simulink model "gm_uz_endat_interface_2023a"  (R2023a)
settings: Solver=FixedStepDiscrete  StartTime=0.0  StopTime=1.3e-3  RelTol=1e-3
undefined symbols (not defined in the file or in its folder): binary_or_gray, bit_sum, delay_first_clk_on_off, endat_clk_divider, endat_encoder_bit_width_multi_turn, endat_encoder_bit_width_single_turn, endat_encoder_number_of_CRC_bits, f_ADC, f_clock, PLL, t_ADC, t_clock
libraries: hdlmdlgenlib x127, simulink x35, hdlsllib x24, simulink_extras x12
(part 1 of 4)
settings Model: Creator=micha  LastModifiedBy=micha
settings SolverCC: AlgebraicLoopSolver=TrustRegion
settings DataIOCC: LimitDataPoints=on  SaveOutput=off  SaveTime=off
settings OptimizationCC: BlockReduction=off  ConditionallyExecuteInputs=off  DefaultParameterBehavior=Inlined  InheritOutputTypeSmallerThanSingle=on  LifeSpan=inf
settings DebuggingCC: AlgebraicLoopMsg=error  ArtificialAlgebraicLoopMsg=none  InheritedTsInSrcMsg=none  SingleTaskRateTransMsg=error  UnconnectedInputMsg=warning  UnconnectedOutputMsg=warning  UnconnectedLineMsg=warning  AllowSymbolicDim=off  StrictBusMsg=ErrorOnBusTreatedAsVector  SFUnexpectedBacktrackingDiag=warning  SFNoUnconditionalDefaultTransitionDiag=warning  SFExecutionAtInitializationDiag=none  ArithmeticOperatorsInVariantConditions=warning
settings HardwareCC: ProdBitPerPointer=32  ProdBitPerSizeT=32  ProdBitPerPtrDiffT=32  ProdLargestAtomicFloat=None  ProdIntDivRoundTo=Undefined  ProdEndianess=Unspecified  ProdWordSize=32  ProdHWDeviceType=ASIC/FPGA->ASIC/FPGA  ProdEqTarget=off
settings ModelReferenceCC: EnableRefExpFcnMdlSchedulingChecks=on
settings SFSimCC: SimUseLocalCustomCode=off  CustomCodeUndefinedFunction=UseInterfaceOnly
settings RTWCC: RTWUseLocalCustomCode=off  DLArmComputeVersion=19.05
settings CodeAppCC: StateflowObjectComments=on
settings GRTTargetCC: TargetLangStandard=C89/C90 (ANSI)
settings ConfigComp: CovScope=ReferencedModels  CovMetricSettings=dw  CovSaveCumulativeToWorkspaceVar=on  CovSaveSingleToWorkspaceVar=on  CovExternalEMLEnable=off  CovSFcnEnable=off

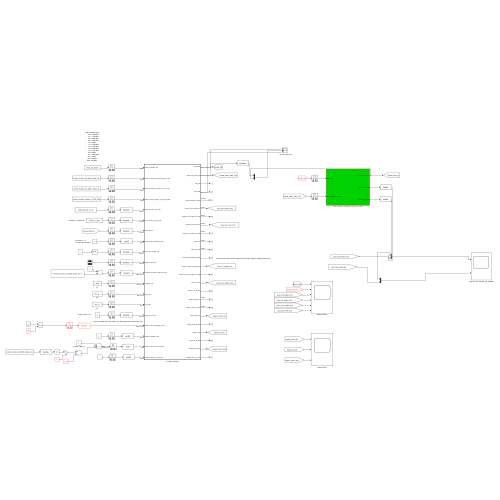
[thumbnail: Simulink's stored preview of the top-level diagram]
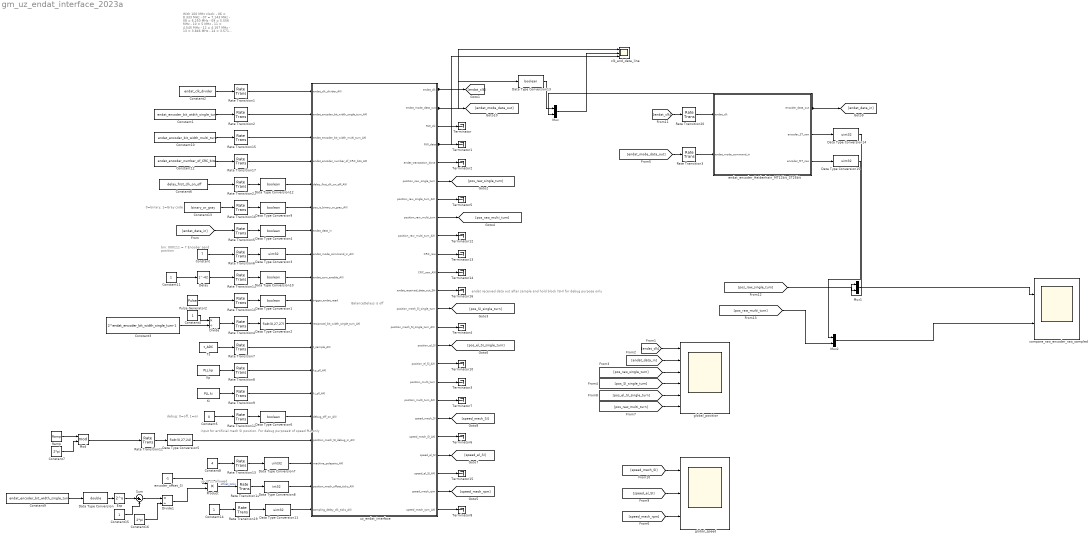
== system gm_uz_endat_interface_2023a ==
  note: 0=binary, 1=Gray code
  note: With 100 MHz clock:
      | -     06 = 8.333 MHz
      | -     07 = 7.143 MHz
      | -     08 = 6.250 MHz
      | -     09 = 5.556 MHz
      | -     10 = 5 MHz
      | -     11 = 4.545 MHz
      | -     12 = 4.167 MHz
      | -     13 = 3.846 MHz
      | -     14 = 3.571 MHz
      | -     25 = 2 MHz
      | -     27 = 1.852 MHz
      | -     50 = 1 MHz
      | -   100 = 500 kHz
      | -   200 = 250 kHz
  note: BalanceDelays is off
  note: debug: 0=off, 1=on
  note: up to 21 allowed
  note: endat received data out after sample and hold block (SH) for debug purpose only
  note: input for artificial mech SI position. For debug purpose# of speed PLL only
  note: bin: 000111 = 7
      | Encoder send position
  Constant : Constant  Value=7  SampleTime=-1
  Constant1 : Constant  Value=endat_encoder_bit_width_single_turn  OutDataTypeStr=uint32  SampleTime=t_clock
  Constant10 : Constant  Value=endat_encoder_bit_width_multi_turn  OutDataTypeStr=uint32  SampleTime=t_clock
  Constant{4,11,14..15} (4 alike) : Constant  SampleTime=t_clock
  Constant12 : Constant  Value=endat_encoder_number_of_CRC_bits  OutDataTypeStr=uint32  SampleTime=t_clock
  Constant13 : Constant  Value=binary_or_gray  OutDataTypeStr=uint32  SampleTime=t_clock
  Constant16 : Constant  Value=2*pi  SampleTime=t_clock
  Constant2 : Constant  Value=endat_clk_divider  OutDataTypeStr=uint32  SampleTime=t_clock
  Constant3 : Constant  Value=2^endat_encoder_bit_width_single_turn-1  OutDataTypeStr=double  SampleTime=t_clock
  Constant5 : Constant  Value=0  SampleTime=t_clock
  Constant6 : Constant  Value=delay_first_clk_on_off  SampleTime=-1
  Constant7 : Constant  Value=2*pi  SampleTime=t_clock
  Constant8 : Constant  Value=4  SampleTime=t_clock
  Constant9 : Constant  Value=endat_encoder_bit_width_single_turn  OutDataTypeStr=uint32  SampleTime=t_clock
  Data Type Conversion : DataTypeConversion  OutDataTypeStr=double  SaturateOnIntegerOverflow=off  RndMeth=Floor
  Data Type Conversion{1,4,6,9..10,12..13} (7 alike) : DataTypeConversion  OutDataTypeStr=boolean  SaturateOnIntegerOverflow=off  RndMeth=Floor
  Data Type Conversion{3,7,11,14..15} (5 alike) : DataTypeConversion  OutDataTypeStr=uint32  SaturateOnIntegerOverflow=off  RndMeth=Floor
  Data Type Conversion2 : DataTypeConversion  OutDataTypeStr=fixdt(0,27,27)  SaturateOnIntegerOverflow=off  RndMeth=Floor
  Data Type Conversion5 : DataTypeConversion  OutDataTypeStr=fixdt(0,27,24)  SaturateOnIntegerOverflow=off  RndMeth=Floor
  Data Type Conversion8 : DataTypeConversion  OutDataTypeStr=int32  SaturateOnIntegerOverflow=off  RndMeth=Floor
  Delay : Delay  DelayLength=42
  Divide : Product  Inputs=*/
  Divide1 : Product  Inputs=*/
  Exp : Math  Operator=2^u
  Ki : Constant  Value=PLL.ki  OutDataTypeStr=fixdt(0,18,0)  SampleTime=-1
  Kp : Constant  Value=PLL.kp  OutDataTypeStr=fixdt(0,18,5)  SampleTime=-1
  Mod : Math  Operator=mod
  Mux : Mux  Inputs=2
  Mux1 : Mux  Inputs=2
  Mux2 : Mux  Inputs=2
  Product : Product
  Pulse Generator2 : DiscretePulseGenerator  Period=f_clock/f_ADC  PulseWidth=0.04*f_clock/f_ADC  PhaseDelay=250  SampleTime=t_clock
  Ramp : simulink/Sources/Ramp  slope=2*pi*100  start=7.5e-5  InitialOutput=0
  Rate Transition{1..21} (21 alike) : RateTransition  OutPortSampleTime=t_clock
  Sum : Sum  Inputs=|+-
  Terminator{,1..8,10,12..16} (15 alike) : Terminator
  Ts : Constant  Value=t_ADC  OutDataTypeStr=fixdt(0,18,24)  SampleTime=-1
  clk_and_data_line : Scope  NumInputPorts=3
  compare_raw_encoder_raw_sampled : Scope  NumInputPorts=2
  encoder_offset_SI : Constant  Value=-1  SampleTime=t_clock
  endat_encoder_Heidenhain_MT12bit_ST25bit : Subsystem
  global_position : Scope  NumInputPorts=6
  global_speed : Scope  NumInputPorts=3
  uz_endat_interface : Subsystem  TreatAsAtomicUnit=on
  wires:
  Data Type Conversion15/1 -> Mux2/1
  Data Type Conversion14/1 -> Mux1/1
  Mux2/1 -> compare_raw_encoder_raw_sampled/2
  Mux1/1 -> compare_raw_encoder_raw_sampled/1
  [pos_raw_multi_turn] -> Mux2/2
  [pos_raw_single_turn] -> Mux1/2
  endat_encoder_Heidenhain_MT12bit_ST25bit/3(encoder_MT_raw) -> Data Type Conversion15/1
  endat_encoder_Heidenhain_MT12bit_ST25bit/2(encoder_ST_raw) -> Data Type Conversion14/1
  Pulse Generator2/1 -> Rate Transition10/1
  Data Type Conversion13/1 -> Mux/1
  Mux/1 -> clk_and_data_line/2
  Rate Transition21/1 -> Data Type Conversion12/1
  Constant6/1 -> Rate Transition21/1
  Data Type Conversion12/1 -> uz_endat_interface/5(delay_first_clk_on_off_AXI)
  Constant/1 -> Rate Transition6/1
  Rate Transition6/1 -> Data Type Conversion3/1
  Data Type Conversion3/1 -> uz_endat_interface/8(endat_mode_command_in_AXI)
  Rate Transition3/1 -> endat_encoder_Heidenhain_MT12bit_ST25bit/2(endat_mode_command_in)
  [endat_mode_data_out] -> Rate Transition3/1
  uz_endat_interface/2(endat_mode_data_out) -> [endat_mode_data_out], Data Type Conversion13/1
  Data Type Conversion/1 -> Exp/1
  Divide1/1 -> Product/2
  Constant16/1 -> Divide1/2
  Sum/1 -> Divide1/1
  Exp/1 -> Sum/1
  Constant15/1 -> Sum/2
  Constant9/1 -> Data Type Conversion/1
  Product/1 -> Rate Transition14/1  "offset_ticks"
  uz_endat_interface/18(position_multi_turn_AXI) -> Terminator7/1
  uz_endat_interface/17(position_multi_turn) -> Terminator3/1
  endat_encoder_Heidenhain_MT12bit_ST25bit/1(encoder_data_out) -> [endat_data_in], Mux/2
  Rate Transition20/1 -> endat_encoder_Heidenhain_MT12bit_ST25bit/1(endat_clk)
  [endat_clk] -> Rate Transition20/1
  Constant14/1 -> Rate Transition19/1
  Rate Transition19/1 -> Data Type Conversion11/1
  Data Type Conversion11/1 -> uz_endat_interface/19(sampling_delay_clk_ticks_AXI)
  [speed_el_SI] -> global_speed/2
  [speed_mech_SI] -> global_speed/1
  [pos_el_SI_single_turn] -> global_position/5
  [pos_raw_multi_turn] -> global_position/6
  [speed_mech_rpm] -> global_speed/3
  Delay/1 -> Rate Transition18/1
  uz_endat_interface/23(speed_mech_rpm) -> [speed_mech_rpm]
  uz_endat_interface/12(endat_received_data_out_SH) -> Terminator16/1
  uz_endat_interface/13(position_mech_SI_single_turn) -> [pos_SI_single_turn]
  [pos_SI_single_turn] -> global_position/4
  [pos_raw_single_turn] -> global_position/3
  uz_endat_interface/6(position_raw_single_turn) -> [pos_raw_single_turn]
  [endat_data_in] -> global_position/2
  [endat_clk] -> global_position/1
  uz_endat_interface/21(speed_el_SI) -> [speed_el_SI]
  uz_endat_interface/22(speed_el_SI_AXI) -> Terminator15/1
  uz_endat_interface/11(CRC_raw_AXI) -> Terminator14/1
  uz_endat_interface/10(CRC_raw) -> Terminator13/1
  uz_endat_interface/9(position_raw_multi_turn_AXI) -> Terminator12/1
  uz_endat_interface/8(position_raw_multi_turn) -> [pos_raw_multi_turn]
  Constant11/1 -> Delay/1
  Rate Transition18/1 -> Data Type Conversion10/1
  Data Type Conversion10/1 -> uz_endat_interface/9(endat_com_enable_AXI)
  Constant12/1 -> Rate Transition17/1
  Rate Transition17/1 -> uz_endat_interface/4(endat_encoder_number_of_CRC_bits_AXI)
  Data Type Conversion9/1 -> uz_endat_interface/6(pos_is_binary_or_gray_AXI)
  Constant13/1 -> Rate Transition16/1
  Rate Transition16/1 -> Data Type Conversion9/1
  Constant10/1 -> Rate Transition15/1
  Rate Transition15/1 -> uz_endat_interface/3(endat_encoder_bit_width_multi_turn_AXI)
  uz_endat_interface/16(position_el_SI_AXI) -> Terminator10/1
  uz_endat_interface/15(position_el_SI) -> [pos_el_SI_single_turn]
  Data Type Conversion8/1 -> uz_endat_interface/18(position_mech_offset_ticks_AXI)
  encoder_offset_SI/1 -> Product/1
  Rate Transition14/1 -> Data Type Conversion8/1
  Constant8/1 -> Rate Transition13/1
  Data Type Conversion7/1 -> uz_endat_interface/17(machine_polepairs_AXI)
  Rate Transition13/1 -> Data Type Conversion7/1
  uz_endat_interface/24(speed_mech_rpm_AXI) -> Terminator8/1
  Constant7/1 -> Mod/2
  Ramp/1 -> Mod/1
  Mod/1 -> Rate Transition11/1
  Constant5/1 -> Rate Transition12/1
  Rate Transition12/1 -> Data Type Conversion6/1
  Data Type Conversion6/1 -> uz_endat_interface/15(debug_off_on_AXI)
  Data Type Conversion5/1 -> uz_endat_interface/16(position_mech_SI_debug_in_AXI)
  Rate Transition11/1 -> Data Type Conversion5/1
  uz_endat_interface/20(speed_mech_SI_AXI) -> Terminator6/1
  uz_endat_interface/19(speed_mech_SI) -> [speed_mech_SI]
  Rate Transition9/1 -> uz_endat_interface/14(ki_pll_AXI)
  Ki/1 -> Rate Transition9/1
  Rate Transition8/1 -> uz_endat_interface/13(kp_pll_AXI)
  Kp/1 -> Rate Transition8/1
  Rate Transition7/1 -> uz_endat_interface/12(t_sample_AXI)
  Ts/1 -> Rate Transition7/1
  uz_endat_interface/14(position_mech_SI_single_turn_AXI) -> Terminator4/1
  Divide/1 -> Rate Transition4/1
  Constant4/1 -> Divide/1
  Data Type Conversion2/1 -> uz_endat_interface/11(reciprocal_bit_width_single_turn_AXI)
  Rate Transition4/1 -> Data Type Conversion2/1
  Constant3/1 -> Divide/2
  Data Type Conversion4/1 -> uz_endat_interface/7(endat_data_in)
  Rate Transition5/1 -> Data Type Conversion4/1
  uz_endat_interface/7(position_raw_single_turn_AXI) -> Terminator5/1
  Data Type Conversion1/1 -> uz_endat_interface/10(trigger_endat_read)
  uz_endat_interface/3(RW_clk) -> Terminator/1
  uz_endat_interface/5(endat_transaction_done) -> Terminator2/1
  uz_endat_interface/4(RW_data) -> Terminator1/1, clk_and_data_line/3
  uz_endat_interface/1(endat_clk) -> [endat_clk], clk_and_data_line/1
  [endat_data_in] -> Rate Transition5/1
  Rate Transition2/1 -> uz_endat_interface/2(endat_encoder_bit_width_single_turn_AXI)
  Constant1/1 -> Rate Transition2/1
  Rate Transition1/1 -> uz_endat_interface/1(endat_clk_divider_AXI)
  Constant2/1 -> Rate Transition1/1
  Rate Transition10/1 -> Data Type Conversion1/1

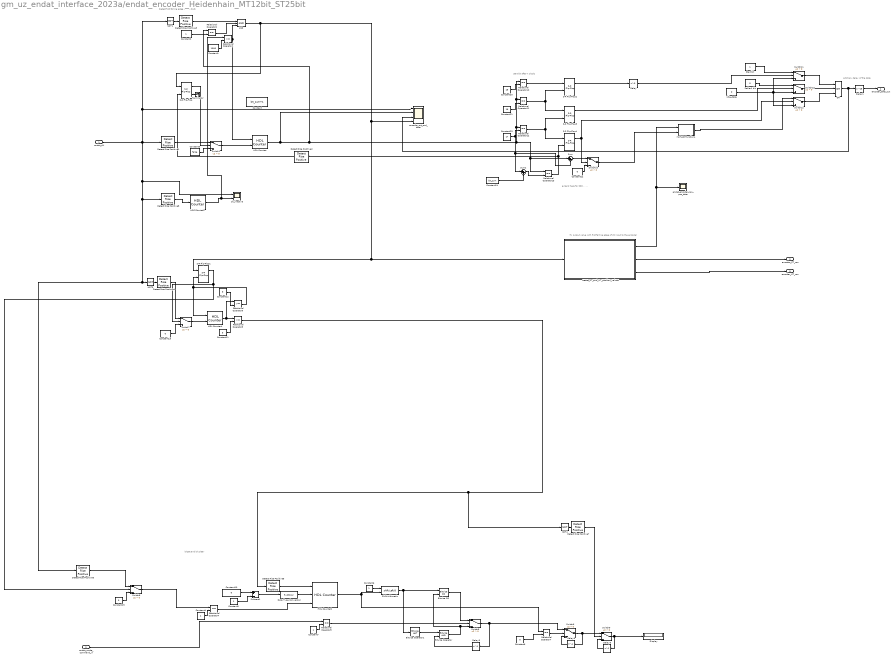
== system gm_uz_endat_interface_2023a/endat_encoder_Heidenhain_MT12bit_ST25bit ==
  note: bitset and bit clear
  note: Detect first falling edge of the clock
  note: arbitrary delay of the data
  note: start bit after n clocks
  note: fix output value with first falling edge of clk input to the encoder
  note: extend here for CRC
      | .
      | .
      | .
      | .
  endat_clk : Inport
  endat_mode_command_in : Inport  Port=2
  AND : Logic  Inputs=3  IconShape=distinctive  AllPortsSameDT=off  OutDataTypeStr=boolean
  Bitwise Operator : simulink/Logic and Bit Operations/Bitwise Operator  logicop=AND  UseBitMask=off  NumInputPorts=2  BitMask=bin2dec('11011001')  BitMaskRealWorld=Stored Integer
  Bitwise Operator1 : simulink/Logic and Bit Operations/Bitwise Operator  logicop=NOT  UseBitMask=off  BitMask=bin2dec('11011001')  BitMaskRealWorld=Stored Integer
  Bitwise OR : simulink/Logic and Bit Operations/Bitwise Operator  logicop=OR  UseBitMask=off  NumInputPorts=2  BitMask=bin2dec('11011001')  BitMaskRealWorld=Stored Integer
      settings: LibrarySourceBlock=|
      | simulink/Quick Insert/Logic and Bit
      | Operations/Bitwise OR
  Constant : Constant  Value=bit_sum+1  SampleTime=t_clock
  Constant1 : Constant  Value=1000  OutDataTypeStr=uint32  SampleTime=t_clock
  Constant10 : Constant  Value=6  OutDataTypeStr=uint32  SampleTime=-1
  Constant11 : Constant  Value=3  OutDataTypeStr=uint32  SampleTime=-1
  Constant12 : Constant  Value=9  OutDataTypeStr=uint32  SampleTime=-1
  Constant13 : Constant  Value=0  OutDataTypeStr=boolean  SampleTime=t_clock
  Constant19 : Constant  Value=0  OutDataTypeStr=boolean  SampleTime=t_clock
  Constant2 : Constant  SampleTime=t_clock
  Constant20 : Constant  Value=15  OutDataTypeStr=uint32  SampleTime=-1
  Constant21 : Constant  Value=16  OutDataTypeStr=uint32  SampleTime=-1
  Constant22 : Constant  Value=0  OutDataTypeStr=uint32  SampleTime=t_clock
  Constant23 : Constant  Value=17  OutDataTypeStr=uint32  SampleTime=-1
  Constant24 : Constant  Value=bit_sum  OutDataTypeStr=uint32  SampleTime=-1
  Constant3 : Constant  Value=false  SampleTime=t_clock
  Constant4 : Constant  OutDataTypeStr=boolean  SampleTime=t_clock
  Constant6 : Constant  OutDataTypeStr=uint64  SampleTime=t_clock
  Constant7 : Constant  OutDataTypeStr=boolean  SampleTime=t_clock
  Constant8 : Constant  Value=0  OutDataTypeStr=uint64  SampleTime=-1
  Constant9 : Constant  OutDataTypeStr=uint32  SampleTime=t_clock
  Data Type Conversion : DataTypeConversion  OutMin=0  OutMax=63  OutDataTypeStr=fixdt(0,6)  SaturateOnIntegerOverflow=off  RndMeth=Floor
  Delay : Delay  DelayLength=0
  Delay1 : Delay  DelayLength=15  SampleTime=t_clock
  Delay5 : Delay  DelayLength=1
  Delay8 : Delay  DelayLength=1
  Delay9 : Delay  DelayLength=1  InitialCondition=0
  Detect Rise Positive{1..8} (8 alike) : simulink/Logic and Bit Operations/Detect Rise Positive  vinit=0  OutDataTypeStr=boolean
  Display : Display
  Fehler1 bit : Constant  Value=0  OutDataTypeStr=boolean  SampleTime=t_clock
  HDL Counter : hdlsllib/Sources/HDL Counter  CountType=Free running  CountInit=1  CountStep=1  CountMax=71  CountFromType=Initial value  CountFrom=1  CountResetPort=on  CountLoadPort=off  CountEnbPort=on  CountDirPort=off  CountHitOutputPort=off  CountDataType=Unsigned  CountWordLen=8  CountFracLen=0  CountSampTime=t_clock
  HDL Counter1 : hdlsllib/Sources/HDL Counter  CountType=Free running  CountInit=0  CountStep=1  CountMax=71  CountFromType=Initial value  CountFrom=0  CountResetPort=on  CountLoadPort=off  CountEnbPort=off  CountDirPort=off  CountHitOutputPort=off  CountDataType=Unsigned  CountWordLen=32  CountFracLen=0  CountSampTime=t_clock
  HDL Counter2 : hdlsllib/Sources/HDL Counter  CountType=Count limited  CountInit=1  CountStep=-1  CountMax=0  CountFromType=Initial value  CountFrom=1  CountResetPort=off  CountLoadPort=on  CountEnbPort=on  CountDirPort=off  CountHitOutputPort=off  CountDataType=Unsigned  CountWordLen=6  CountFracLen=0  CountSampTime=1
  HDL Counter4 : hdlsllib/Sources/HDL Counter  CountType=Free running  CountInit=0  CountStep=1  CountMax=4095  CountFromType=Initial value  CountFrom=0  CountResetPort=on  CountLoadPort=off  CountEnbPort=on  CountDirPort=off  CountHitOutputPort=off  CountDataType=Unsigned  CountWordLen=8  CountFracLen=0  CountSampTime=1
  MATLAB Function4 : MATLAB Function  TreatAsAtomicUnit=on
  NOT1 : Logic  Operator=NOT  IconShape=distinctive  AllPortsSameDT=off  OutDataTypeStr=boolean
  NOT3 : Logic  Operator=NOT  IconShape=distinctive  AllPortsSameDT=off  OutDataTypeStr=boolean
  NOT4 : Logic  Operator=NOT  IconShape=distinctive  AllPortsSameDT=off  OutDataTypeStr=boolean
  OR : Logic  Operator=OR  Inputs=3  IconShape=distinctive  AllPortsSameDT=off  OutDataTypeStr=boolean
  Relational Operator1 : RelationalOperator  OutDataTypeStr=boolean  RndMeth=Simplest  InputSameDT=off
  Relational Operator{2,4..5,7,10..13} (8 alike) : RelationalOperator  Operator===  OutDataTypeStr=boolean  RndMeth=Simplest  InputSameDT=off
  Relational Operator8 : RelationalOperator  OutDataTypeStr=boolean  RndMeth=Simplest  InputSameDT=off
  Relational Operator9 : RelationalOperator  OutDataTypeStr=boolean  RndMeth=Simplest  InputSameDT=off
  S-R Flip-Flop{,1..4} (5 alike) : simulink_extras/Flip Flops/S-R Flip-Flop  initial_condition=0
  Shift Arithmetic : ArithShift  BitShiftNumberSource=Input port  BitShiftNumber=8  BitShiftDirection=Left
      settings: InputPortMap=u0,p1
  Start bit : Constant  OutDataTypeStr=boolean  SampleTime=t_clock
  Subtract1 : Sum  Inputs=+-  OutDataTypeStr=uint32
  Sum : Sum  Inputs=|+-
  Sum2 : Sum  Inputs=|++
  Switch{1,5..13} (10 alike) : Switch  Criteria=u2 > Threshold  SaturateOnIntegerOverflow=off  InputSameDT=off
  Terminator : Terminator
  clk_inactive : Scope  NumInputPorts=2
  create_ST_and_MT_position_values : Subsystem
  encoder_cnt_and_data : Scope  NumInputPorts=4
  endat_encoder_raw_pos_data : Scope
  idle_state : Constant  Value=0  OutDataTypeStr=boolean  SampleTime=t_clock
  encoder_data_out : Outport
  encoder_ST_raw : Outport  Port=2
  encoder_MT_raw : Outport  Port=3
  wires:
  Relational Operator1/1 -> HDL Counter/1, AND/3
  Delay/1 -> Switch11/2
  create_ST_and_MT_position_values/3(encoder_MT_raw) -> encoder_MT_raw/1
  create_ST_and_MT_position_values/2(encoder_ST_raw) -> encoder_ST_raw/1
  S-R Flip-Flop/2 -> Terminator/1
  Constant3/1 -> Switch1/3
  Constant1/1 -> Relational Operator1/2
  HDL Counter1/1 -> clk_inactive/2, Relational Operator1/1
  Detect Rise Positive8/1 -> HDL Counter1/1
  endat_clk/1 -> Detect Rise Positive1/1, NOT3/1, Detect Rise Positive6/1, Detect Rise Positive8/1, clk_inactive/1, encoder_cnt_and_data/1, NOT1/1
  Detect Rise Positive2/1 -> S-R Flip-Flop/2
  Switch1/1 -> HDL Counter/2
  Detect Rise Positive1/1 -> Switch1/1
  S-R Flip-Flop/1 -> Switch1/2
  HDL Counter/1 -> Relational Operator2/1, Relational Operator13/1, Sum/1, Relational Operator12/1, Relational Operator11/1, Relational Operator10/1, encoder_cnt_and_data/2
  create_ST_and_MT_position_values/1(pos_data) -> endat_encoder_raw_pos_data/1, MATLAB Function4/1(u)
  Relational Operator13/1 -> Detect Rise Positive2/1, S-R Flip-Flop4/2
  Sum/1 -> Switch10/1
  Constant24/1 -> Sum2/2
  Sum2/1 -> Relational Operator13/2
  Switch10/1 -> MATLAB Function4/2(cnt)
  S-R Flip-Flop4/1 -> Switch10/2, Switch12/2
  Switch13/1 -> OR/2
  Switch12/1 -> OR/3
  OR/1 -> Delay1/1, encoder_cnt_and_data/3
  idle_state/1 -> Switch11/3, Switch13/3, Switch12/3
  Relational Operator12/1 -> S-R Flip-Flop3/2, S-R Flip-Flop4/1
  Constant23/1 -> Relational Operator12/2, Sum/2, Sum2/1
  S-R Flip-Flop3/1 -> Switch13/2
  Fehler1 bit/1 -> Switch13/1
  Start bit/1 -> Switch11/1
  Constant22/1 -> Switch10/3
  Relational Operator11/1 -> S-R Flip-Flop2/2, S-R Flip-Flop3/1
  Constant21/1 -> Relational Operator11/2
  Switch11/1 -> OR/1
  S-R Flip-Flop2/1 -> Delay/1
  Relational Operator10/1 -> S-R Flip-Flop2/1
  Constant20/1 -> Relational Operator10/2
  Detect Rise Positive7/1 -> Switch9/2
  NOT4/1 -> Detect Rise Positive7/1
  Switch9/1 -> Display/1, Delay9/1
  Delay9/1 -> Switch9/3
  S-R Flip-Flop1/1 -> Switch7/2, Switch8/2
  Constant19/1 -> Switch8/3
  Switch8/1 -> Relational Operator4/1
  Detect Rise Positive6/1 -> Switch8/1
  NOT3/1 -> Detect Rise Positive4/1
  Constant13/1 -> Switch7/3
  Switch7/1 -> HDL Counter4/2
  Relational Operator9/1 -> S-R Flip-Flop1/2, HDL Counter4/1
  Constant12/1 -> Relational Operator9/2
  Constant11/1 -> Relational Operator8/2
  HDL Counter4/1 -> Relational Operator8/1, Relational Operator9/1  "MT_bin"
  Relational Operator8/1 -> NOT4/1, Detect Rise Positive5/1
  Constant6/1 -> Shift Arithmetic/1
  Relational Operator4/1 -> HDL Counter2/3
  Detect Rise Positive5/1 -> HDL Counter2/1
  Relational Operator5/1 -> Switch5/2
  HDL Counter2/1 -> Relational Operator7/1, Shift Arithmetic/2  "pos"
  Delay5/1 -> Bitwise Operator/2
  Constant10/1 -> Subtract1/1  "bit_sum"
  Constant7/1 -> Relational Operator5/2
  Constant4/1 -> Relational Operator4/2
  Constant8/1 -> Relational Operator7/2
  Switch6/1 -> Switch9/1, Delay8/1
  Bitwise Operator1/1 -> Bitwise Operator/1  "mask_clear"
  Switch5/1 -> Delay5/1, Switch6/1
  Shift Arithmetic/1 -> Bitwise Operator1/1, Bitwise OR/1  "mask_set"
  AND/1 -> encoder_cnt_and_data/4, create_ST_and_MT_position_values/1(first_falling_edge_trigger), S-R Flip-Flop1/1, S-R Flip-Flop/1
  Constant9/1 -> Subtract1/2
  Bitwise Operator/1 -> Bitwise OR/2, Switch5/3
  Bitwise OR/1 -> Switch5/1
  endat_mode_command_in/1 -> Relational Operator5/1
  Subtract1/1 -> Data Type Conversion/1  "pos"
  Relational Operator7/1 -> Switch6/2
  Delay8/1 -> Switch6/3
  Data Type Conversion/1 -> HDL Counter2/2
  Detect Rise Positive4/1 -> Switch7/1
  MATLAB Function4/1(y) -> Switch12/1
  Delay1/1 -> encoder_data_out/1
  Detect Rise Positive3/1 -> AND/1
  NOT1/1 -> Detect Rise Positive3/1
  Constant2/1 -> Relational Operator2/2
  Relational Operator2/1 -> AND/2

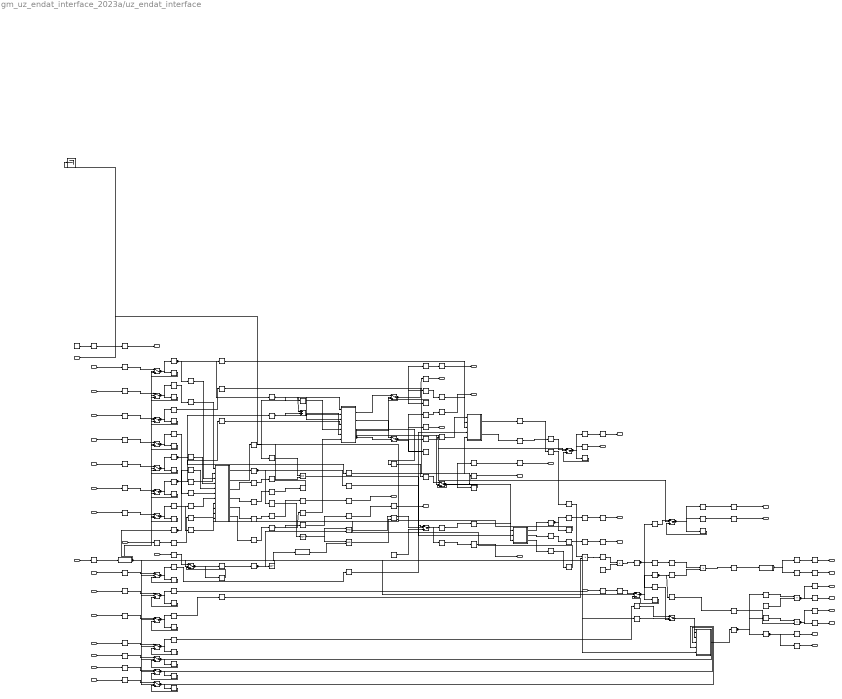
== system gm_uz_endat_interface_2023a/uz_endat_interface ==
  note: raw position with encoder offset and aligned wrap for ST and MT position
  note: Processing of raw position data
  note: mech speed SI to el speed SI
  note: decode position and slice data
  note: mech speed SI to el speed SI
  note: SI electrical position
  note: mech speed SI to mech speed RPM
  note: SI mech position to mech speed SI
  note: Acquisition of raw position data from the EnDat absolute encoder
  note: ST mech position to SI mech position
  note: pull clk high when disabled
  note: enable logic for clock: turns on and off clk only between transmissions
  note: Set data transceiver to send/receive mode and set mode command bits with respective clock pulses
  endat_clk_divider_AXI : Inport  OutDataTypeStr=uint32  PortDimensions=1  SampleTime=1e-08
  endat_encoder_bit_width_single_turn_AXI : Inport  Port=2  OutDataTypeStr=uint32  PortDimensions=1  SampleTime=1e-08
  endat_encoder_bit_width_multi_turn_AXI : Inport  Port=3  OutDataTypeStr=uint32  PortDimensions=1  SampleTime=1e-08
  endat_encoder_number_of_CRC_bits_AXI : Inport  Port=4  OutDataTypeStr=uint32  PortDimensions=1  SampleTime=1e-08
  delay_first_clk_on_off_AXI : Inport  Port=5  OutDataTypeStr=boolean  PortDimensions=1  SampleTime=1e-08
  pos_is_binary_or_gray_AXI : Inport  Port=6  OutDataTypeStr=boolean  PortDimensions=1  SampleTime=1e-08
  endat_data_in : Inport  Port=7  OutDataTypeStr=boolean  PortDimensions=1  SampleTime=1e-08
  endat_mode_command_in_AXI : Inport  Port=8  OutDataTypeStr=uint32  PortDimensions=1  SampleTime=1e-08
  endat_com_enable_AXI : Inport  Port=9  OutDataTypeStr=boolean  PortDimensions=1  SampleTime=1e-08
  trigger_endat_read : Inport  Port=10  OutDataTypeStr=boolean  PortDimensions=1  SampleTime=1e-08
  reciprocal_bit_width_single_turn_AXI : Inport  Port=11  OutDataTypeStr=fixdt(0, 27, 27)  PortDimensions=1  SampleTime=1e-08
  t_sample_AXI : Inport  Port=12  OutDataTypeStr=fixdt(0, 18, 24)  PortDimensions=1  SampleTime=1e-08
  kp_pll_AXI : Inport  Port=13  OutDataTypeStr=fixdt(0, 18, 5)  PortDimensions=1  SampleTime=1e-08
  ki_pll_AXI : Inport  Port=14  OutDataTypeStr=fixdt(0, 18, 0)  PortDimensions=1  SampleTime=1e-08
  debug_off_on_AXI : Inport  Port=15  OutDataTypeStr=boolean  PortDimensions=1  SampleTime=1e-08
  position_mech_SI_debug_in_AXI : Inport  Port=16  OutDataTypeStr=fixdt(0, 27, 24)  PortDimensions=1  SampleTime=1e-08
  machine_polepairs_AXI : Inport  Port=17  OutDataTypeStr=uint32  PortDimensions=1  SampleTime=1e-08
  position_mech_offset_ticks_AXI : Inport  Port=18  OutDataTypeStr=int32  PortDimensions=1  SampleTime=1e-08
  sampling_delay_clk_ticks_AXI : Inport  Port=19  OutDataTypeStr=uint32  PortDimensions=1  SampleTime=1e-08
  AND : Logic  AllPortsSameDT=off  OutDataTypeStr=boolean  SampleTime=1e-08
  AND1 : Logic  AllPortsSameDT=off  OutDataTypeStr=boolean  SampleTime=1e-08
  Constant : Constant  Value=6.283172607421875  OutDataTypeStr=fixdt(0, 18, 15)  SampleTime=1e-08
  Constant1 : Constant  OutDataTypeStr=boolean  SampleTime=1e-08
  Constant4 : Constant  Value=9.54931640625  OutDataTypeStr=fixdt(0, 18, 14)  SampleTime=1e-08
  Constant5 : Constant  OutDataTypeStr=boolean  SampleTime=1e-08
  Data Type Conversion : DataTypeConversion  OutDataTypeStr=uint8  SampleTime=1e-08  SaturateOnIntegerOverflow=off  RndMeth=Floor
  Data Type Conversion1 : DataTypeConversion  OutDataTypeStr=int32  SampleTime=1e-08  SaturateOnIntegerOverflow=off  RndMeth=Floor
  Delay{,4..8,10..11,13..20,22,24,26..27,29,33..34,37,39..43,48,50..52,54..58,60,129} (40 alike) : Delay  DelayLength=double(1)  InitialCondition=0  SampleTime=1e-08
  Delay1 : Delay  DelayLength=double(1)  InitialCondition=25  SampleTime=1e-08
  Delay{2..3,9,12,21,23,25,28,30,32,36,38,45,49,53,59,61..64} (20 alike) : Delay  DelayLength=double(2)  InitialCondition=0  SampleTime=1e-08
  Delay127 : Delay  DelayLength=double(1)  InitialCondition=1  SampleTime=1e-08
  Delay31 : Delay  DelayLength=double(1)  InitialCondition=25  SampleTime=1e-08
  Delay35 : Delay  DelayLength=double(1)  InitialCondition=1  SampleTime=1e-08
  Delay44 : Delay  DelayLength=double(1)  InitialCondition=12  SampleTime=1e-08
  Detect Rise Positive : simulink/Logic and Bit Operations/Detect Rise Positive  vinit=0  OutDataTypeStr=boolean
  Detect Rise Positive1 : simulink/Logic and Bit Operations/Detect Rise Positive  vinit=0  OutDataTypeStr=boolean
  From{,1..14,16,18..47} (46 alike) : hdlmdlgenlib/Buffer
  Goto{,1..15,17..32} (32 alike) : hdlmdlgenlib/Buffer
  NOT : Logic  Operator=NOT  Inputs=1  AllPortsSameDT=off  OutDataTypeStr=boolean  SampleTime=1e-08
  NOT1 : Logic  Operator=NOT  Inputs=1  AllPortsSameDT=off  OutDataTypeStr=boolean  SampleTime=1e-08
  OR : Logic  Operator=OR  AllPortsSameDT=off  OutDataTypeStr=boolean  SampleTime=1e-08
  Product : Product  Inputs=**  OutDataTypeStr=fixdt(0, 27, 24)  SampleTime=1e-08
  Product1 : Product  Inputs=**  OutDataTypeStr=fixdt(1, 27, 12)  SampleTime=1e-08
  Product2 : Product  Inputs=**  OutDataTypeStr=fixdt(1, 27, 12)  SampleTime=1e-08
  Product4 : Product  Inputs=**  OutDataTypeStr=fixdt(0, 27, 20)  SampleTime=1e-08
  Product7 : Product  Inputs=**  OutDataTypeStr=fixdt(0, 27, 24)  SampleTime=1e-08
  RW_data_and_mode_command_control : Subsystem
  S-R Flip-Flop1 : simulink_extras/Flip Flops/S-R Flip-Flop  initial_condition=0
  S-R Flip-Flop1_inst_term1 : Terminator
  Sum2 : Sum  AccumDataTypeStr=fixdt(0, 33, 0)  OutDataTypeStr=int32  SampleTime=1e-08
  Switch{1,5..6,13,15..16,19..21,31} (10 alike) : Switch  Criteria=u2 > Threshold  Threshold=double(0)  OutDataTypeStr=uint32  SampleTime=1e-08  SaturateOnIntegerOverflow=off  InputSameDT=off
  Switch10 : Switch  Criteria=u2 > Threshold  Threshold=double(0)  OutDataTypeStr=fixdt(0, 27, 24)  SampleTime=1e-08  SaturateOnIntegerOverflow=off  InputSameDT=off
  Switch11 : Switch  Criteria=u2 > Threshold  Threshold=double(0)  OutDataTypeStr=uint8  SampleTime=1e-08  SaturateOnIntegerOverflow=off  InputSameDT=off
  Switch12 : Switch  Criteria=u2 > Threshold  Threshold=double(0)  OutDataTypeStr=int32  SampleTime=1e-08  SaturateOnIntegerOverflow=off  InputSameDT=off
  Switch{8,17..18,23} (4 alike) : Switch  Criteria=u2 > Threshold  Threshold=double(0)  OutDataTypeStr=boolean  SampleTime=1e-08  SaturateOnIntegerOverflow=off  InputSameDT=off
  Switch2 : Switch  Criteria=u2 > Threshold  Threshold=double(0)  OutDataTypeStr=fixdt(0, 27, 27)  SampleTime=1e-08  SaturateOnIntegerOverflow=off  InputSameDT=off
  Switch22 : Switch  Criteria=u2 > Threshold  Threshold=double(0)  OutDataTypeStr=fixdt(0, 27, 24)  SampleTime=1e-08  SaturateOnIntegerOverflow=off  InputSameDT=off
  Switch3 : Switch  Criteria=u2 > Threshold  Threshold=double(0)  OutDataTypeStr=fixdt(0, 18, 24)  SampleTime=1e-08  SaturateOnIntegerOverflow=off  InputSameDT=off
  Switch4 : Switch  Criteria=u2 > Threshold  Threshold=double(0)  OutDataTypeStr=fixdt(0, 18, 5)  SampleTime=1e-08  SaturateOnIntegerOverflow=off  InputSameDT=off
  Switch7 : Switch  Criteria=u2 > Threshold  Threshold=double(0)  OutDataTypeStr=fixdt(0, 18, 0)  SampleTime=1e-08  SaturateOnIntegerOverflow=off  InputSameDT=off
  Switch9 : Switch  Criteria=u2 > Threshold  Threshold=double(0)  OutDataTypeStr=fixdt(0, 27, 24)  SampleTime=1e-08  SaturateOnIntegerOverflow=off  InputSameDT=off
  delayMatch{,1..18} (19 alike) : Delay  DelayLength=double(1)  InitialCondition=0  SampleTime=1e-08
  pos_is_binary_or_gray_AXI_term5 : Terminator
  position_to_speed_pll : Subsystem
  serial_communication : Subsystem
  set_offset_to_raw_position_and_wrap : Subsystem
  slice_position_and_CRC : Subsystem
  wrap_2pi : Subsystem
  endat_clk : Outport  SampleTime=1e-08
  endat_mode_data_out : Outport  Port=2  SampleTime=1e-08
  RW_clk : Outport  Port=3  SampleTime=1e-08
  RW_data : Outport  Port=4  SampleTime=1e-08
  endat_transaction_done : Outport  Port=5  OutDataTypeStr=boolean  SampleTime=1e-08  LockScale=on
  position_raw_single_turn : Outport  Port=6  OutDataTypeStr=uint32  SampleTime=1e-08  LockScale=on
  position_raw_single_turn_AXI : Outport  Port=7  OutDataTypeStr=uint32  SampleTime=1e-08  LockScale=on
  position_raw_multi_turn : Outport  Port=8  OutDataTypeStr=uint32  SampleTime=1e-08  LockScale=on
  position_raw_multi_turn_AXI : Outport  Port=9  OutDataTypeStr=uint32  SampleTime=1e-08  LockScale=on
  CRC_raw : Outport  Port=10  OutDataTypeStr=uint32  SampleTime=1e-08  LockScale=on
  CRC_raw_AXI : Outport  Port=11  OutDataTypeStr=uint32  SampleTime=1e-08  LockScale=on
  endat_received_data_out_SH : Outport  Port=12  SampleTime=1e-08
  position_mech_SI_single_turn : Outport  Port=13  SampleTime=1e-08
  position_mech_SI_single_turn_AXI : Outport  Port=14  SampleTime=1e-08
  position_el_SI : Outport  Port=15  SampleTime=1e-08
  position_el_SI_AXI : Outport  Port=16  SampleTime=1e-08
  position_multi_turn : Outport  Port=17  OutDataTypeStr=uint32  SampleTime=1e-08  LockScale=on
  position_multi_turn_AXI : Outport  Port=18  OutDataTypeStr=uint32  SampleTime=1e-08  LockScale=on
  speed_mech_SI : Outport  Port=19  SampleTime=1e-08
  speed_mech_SI_AXI : Outport  Port=20  SampleTime=1e-08
  speed_el_SI : Outport  Port=21  SampleTime=1e-08
  speed_el_SI_AXI : Outport  Port=22  SampleTime=1e-08
  speed_mech_rpm : Outport  Port=23  SampleTime=1e-08
  speed_mech_rpm_AXI : Outport  Port=24  SampleTime=1e-08
  wires:
  endat_clk_divider_AXI/1 -> Delay64/1
  endat_encoder_bit_width_single_turn_AXI/1 -> Delay2/1
  endat_encoder_bit_width_multi_turn_AXI/1 -> Delay45/1
  endat_encoder_number_of_CRC_bits_AXI/1 -> Delay49/1
  delay_first_clk_on_off_AXI/1 -> Delay61/1
  pos_is_binary_or_gray_AXI/1 -> pos_is_binary_or_gray_AXI_term5/1
  endat_data_in/1 -> Delay3/1
  endat_mode_command_in_AXI/1 -> Delay59/1
  endat_com_enable_AXI/1 -> Delay53/1
  trigger_endat_read/1 -> Delay32/1
  reciprocal_bit_width_single_turn_AXI/1 -> Delay9/1
  t_sample_AXI/1 -> Delay21/1
  kp_pll_AXI/1 -> Delay23/1
  ki_pll_AXI/1 -> Delay25/1
  debug_off_on_AXI/1 -> Delay28/1
  position_mech_SI_debug_in_AXI/1 -> Delay30/1
  machine_polepairs_AXI/1 -> Delay36/1
  position_mech_offset_ticks_AXI/1 -> Delay38/1
  sampling_delay_clk_ticks_AXI/1 -> Delay12/1
  Constant/1 -> Product7/2
  Constant1/1 -> Delay4/1
  Constant4/1 -> Product1/2
  Constant5/1 -> Switch17/3
  Data Type Conversion/1 -> Switch11/1
  Data Type Conversion1/1 -> slice_position_and_CRC/5(shift_val_mt)
  Delay/1 -> Product/1
  delayMatch13/1 -> position_mech_SI_single_turn/1
  delayMatch14/1 -> position_mech_SI_single_turn_AXI/1
  Delay12/1 -> Switch20/1
  delayMatch1/1 -> endat_clk/1
  delayMatch5/1 -> endat_transaction_done/1
  delayMatch7/1 -> position_raw_single_turn_AXI/1
  delayMatch12/1 -> endat_received_data_out_SH/1
  Delay18/1 -> speed_mech_SI_AXI/1
  Delay19/1 -> speed_mech_SI/1
  Delay2/1 -> Switch1/1
  Delay21/1 -> Switch3/1
  Delay23/1 -> Switch4/1
  Delay25/1 -> Switch7/1
  Delay26/1 -> Product7/1
  Delay28/1 -> Switch8/1
  Delay3/1 -> Goto3/1
  Delay30/1 -> Switch10/1
  Delay32/1 -> Detect Rise Positive1/1
  Delay33/1 -> speed_mech_rpm/1
  Delay34/1 -> speed_mech_rpm_AXI/1
  Delay36/1 -> Data Type Conversion/1
  Delay38/1 -> Switch12/1
  Delay39/1 -> Product4/1
  delayMatch3/1 -> RW_clk/1
  delayMatch15/1 -> position_el_SI/1
  delayMatch18/1 -> position_multi_turn_AXI/1
  delayMatch16/1 -> position_el_SI_AXI/1
  Delay43/1 -> wrap_2pi/1(input)
  Delay45/1 -> Switch13/1
  Delay49/1 -> Switch15/1
  delayMatch9/1 -> position_raw_multi_turn_AXI/1
  Delay53/1 -> Switch18/1
  delayMatch11/1 -> CRC_raw_AXI/1
  Delay56/1 -> speed_el_SI/1
  Delay57/1 -> speed_el_SI_AXI/1
  Delay59/1 -> Switch5/1
  delayMatch2/1 -> endat_mode_data_out/1
  Delay61/1 -> Switch23/1
  Delay62/1 -> Goto17/1
  Delay63/1 -> Goto21/1
  Delay64/1 -> Switch31/1
  delayMatch4/1 -> RW_data/1
  Delay9/1 -> Switch2/1
  Detect Rise Positive/1 -> AND1/2
  Detect Rise Positive1/1 -> Goto22/1, position_to_speed_pll/5(Trigger), Switch31/2, Switch1/2, Switch13/2, Switch11/2, Switch18/2, Switch5/2, Switch15/2, Switch23/2, Switch20/2, Switch12/2, Switch2/2, Switch10/2, Switch8/2, Switch3/2, Switch4/2, Switch7/2
  From/1 -> Delay129/1
  From1/1 -> serial_communication/6(delay_first_clk_on_off)
  From10/1 -> Delay7/1
  From11/1 -> Switch9/2
  From12/1 -> Switch21/1
  From13/1 -> Switch9/1
  From14/1 -> Product1/1
  From16/1 -> Product4/2
  From18/1 -> slice_position_and_CRC/1(data)
  From19/1 -> Switch9/3
  From2/1 -> Delay/1
  From20/1 -> set_offset_to_raw_position_and_wrap/1(mt_raw)
  From21/1 -> Switch22/1
  From22/1 -> Delay39/1
  From23/1 -> serial_communication/3(bit_width_single_turn)
  From24/1 -> serial_communication/4(bit_width_multi_turn)
  From25/1 -> serial_communication/5(bit_width_CRC)
  From27/1 -> NOT1/1, AND/2
  From29/1 -> Delay17/1
  From3/1 -> Delay19/1, Delay18/1
  From30/1 -> Switch19/1
  From31/1 -> Product2/1
  delayMatch/1 -> Product2/2
  From34/1 -> RW_data_and_mode_command_control/3(endat_mode_command)
  From35/1 -> Sum2/2, slice_position_and_CRC/2(bit_width_mt)
  From36/1 -> Sum2/1, Data Type Conversion1/1, slice_position_and_CRC/3(bit_width_st)
  From37/1 -> slice_position_and_CRC/4(bit_width_CRC)
  From38/1 -> serial_communication/2(endat_clk_reset)
  From39/1 -> serial_communication/7(trigger_endat)
  From4/1 -> serial_communication/1(endat_clk_divider)
  From41/1 -> Delay6/1
  From42/1 -> set_offset_to_raw_position_and_wrap/3(st_raw)
  From43/1 -> set_offset_to_raw_position_and_wrap/5(n1)
  From44/1 -> set_offset_to_raw_position_and_wrap/2(n)
  From45/1 -> set_offset_to_raw_position_and_wrap/4(In4)
  From6/1 -> Product/2
  From7/1 -> serial_communication/8(endat_data_in)
  From8/1 -> slice_position_and_CRC/7(trigger)
  From9/1 -> serial_communication/9(sampling_delay_clk_ticks)
  NOT1/1 -> Detect Rise Positive/1
  Product/1 -> Delay26/1
  Product1/1 -> Delay34/1, Delay33/1
  Product2/1 -> Delay57/1, Delay56/1
  Product4/1 -> Delay43/1
  Product7/1 -> Goto14/1
  RW_data_and_mode_command_control/2(endat_mode_data_out) -> Goto31/1
  S-R Flip-Flop1/2 -> S-R Flip-Flop1_inst_term1/1
  Sum2/1 -> slice_position_and_CRC/6(shift_val_CRC)
  Switch1/1 -> Goto/1, Delay1/1
  Switch10/1 -> Goto10/1, Delay29/1
  Switch11/1 -> Goto11/1, Delay35/1
  Switch12/1 -> Goto27/1, Delay37/1
  Switch13/1 -> Goto15/1, Delay44/1
  Switch15/1 -> Goto9/1, Delay48/1
  delayMatch8/1 -> position_raw_multi_turn/1
  Switch17/1 -> Delay127/1, Goto30/1
  Switch18/1 -> Goto18/1, Delay52/1
  delayMatch10/1 -> CRC_raw/1
  Switch2/1 -> Goto5/1, Delay8/1
  Switch20/1 -> Goto25/1, Delay5/1
  delayMatch17/1 -> position_multi_turn/1
  Switch22/1 -> Delay11/1, Delay10/1, Delay58/1
  Switch23/1 -> Goto2/1, Delay60/1
  Switch3/1 -> position_to_speed_pll/2(t_sample), Delay20/1
  Switch31/1 -> Goto7/1, Delay31/1
  Switch4/1 -> position_to_speed_pll/3(kp_pll), Delay22/1
  Switch5/1 -> Goto1/1, Delay14/1
  delayMatch6/1 -> position_raw_single_turn/1
  Switch7/1 -> position_to_speed_pll/4(ki_pll), Delay24/1
  Switch8/1 -> Goto8/1, Delay27/1
  Switch9/1 -> position_to_speed_pll/1(position_mech_SI)
  position_to_speed_pll/1(speed_mech_SI) -> Goto12/1
  serial_communication/4(endat_data_raw) -> Delay63/1
  serial_communication/5(endat_data_SH) -> Goto19/1
  serial_communication/6(endat_transaction_done) -> Delay62/1
  set_offset_to_raw_position_and_wrap/1(st_raw_with_offset_and_wrapped) -> Goto29/1
  set_offset_to_raw_position_and_wrap/2(mt_raw_with_offset_and_wrapped) -> Goto28/1
  slice_position_and_CRC/1(pos_raw_st) -> Switch6/1
  slice_position_and_CRC/2(pos_raw_mt) -> Switch16/1
  slice_position_and_CRC/3(raw_CRC) -> Goto20/1
  slice_position_and_CRC/4(slicing_done) -> Switch6/2, Switch16/2, Switch19/2, Switch22/2, Switch21/2
  wrap_2pi/1(output) -> Delay42/1, Delay40/1
  Goto17/1 -> From8/1, From/1
  Goto2/1 -> From1/1
  Goto13/1 -> From10/1, From47/1
  Goto8/1 -> From11/1
  Goto28/1 -> From12/1
  Goto10/1 -> From13/1
  Goto12/1 -> From31/1, From3/1, From14/1
  Goto11/1 -> From32/1, From16/1
  Goto21/1 -> From18/1
  Goto14/1 -> From22/1, From21/1, From19/1
  Goto29/1 -> From2/1
  Goto26/1 -> From20/1
  Goto/1 -> From44/1, From36/1, From23/1
  Goto15/1 -> From43/1, From35/1, From24/1
  Goto9/1 -> From37/1, From25/1
  Goto18/1 -> From27/1
  Goto19/1 -> From29/1
  Goto20/1 -> From30/1
  Goto1/1 -> From34/1
  Goto22/1 -> From39/1, From38/1
  Goto7/1 -> From4/1
  Goto31/1 -> From41/1
  Goto4/1 -> From42/1
  Goto27/1 -> From45/1
  Goto5/1 -> From6/1
  Goto3/1 -> From7/1
  Goto25/1 -> From9/1
  From32/1 -> delayMatch/1
  Delay127/1 -> delayMatch1/1
  Delay6/1 -> delayMatch2/1
  Delay4/1 -> delayMatch3/1
  Delay7/1 -> delayMatch4/1
  Delay129/1 -> delayMatch5/1
  Switch6/1 -> delayMatch6/1, Goto4/1, Delay16/1, Delay15/1
  Delay16/1 -> delayMatch7/1
  Switch16/1 -> delayMatch8/1, Goto26/1, Delay51/1, Delay50/1
  Delay51/1 -> delayMatch9/1
  Switch19/1 -> delayMatch10/1, Delay55/1, Delay54/1
  Delay55/1 -> delayMatch11/1
  Delay17/1 -> delayMatch12/1
  Delay10/1 -> delayMatch13/1
  Delay11/1 -> delayMatch14/1
  Delay40/1 -> delayMatch15/1
  Delay42/1 -> delayMatch16/1
  Switch21/1 -> delayMatch17/1, Delay41/1, Delay13/1
  Delay41/1 -> delayMatch18/1
  Delay24/1 -> Switch7/3
  Delay31/1 -> Switch31/3
  Delay1/1 -> Switch1/3
  Delay44/1 -> Switch13/3
  Delay48/1 -> Switch15/3
  Delay60/1 -> Switch23/3
  Delay5/1 -> Switch20/3
  Delay52/1 -> Switch18/3
  Delay14/1 -> Switch5/3
  S-R Flip-Flop1/1 -> Switch17/2
  From33/1 -> RW_data_and_mode_command_control/1(endat_clk)
  RW_data_and_mode_command_control/1(RW_data) -> Goto13/1
  RW_data_and_mode_command_control/3(poll_for_start_bit) -> Goto32/1
  From47/1 -> serial_communication/10(RW_data)
  serial_communication/1(endat_clk) -> Goto24/1
  serial_communication/2(endat_clk_enb_out) -> Goto6/1
  serial_communication/3(endat_clk_idle_levels) -> Goto23/1
  Goto30/1 -> From33/1
  Goto23/1 -> From40/1
  From40/1 -> OR/2
  Goto24/1 -> From5/1
  From5/1 -> OR/1
  OR/1 -> Switch17/1
  From26/1 -> RW_data_and_mode_command_control/2(endat_clk_enable)
  AND1/1 -> S-R Flip-Flop1/2
  AND/1 -> S-R Flip-Flop1/1
  Goto6/1 -> From28/1, From26/1
  From28/1 -> NOT/1
  NOT/1 -> AND1/1, AND/1
  From46/1 -> serial_communication/11(poll_for_start_bit)
  Goto32/1 -> From46/1
  Delay15/1 -> Switch6/3
  Delay50/1 -> Switch16/3
  Delay54/1 -> Switch19/3
  Delay37/1 -> Switch12/3
  Delay8/1 -> Switch2/3
  Delay58/1 -> Switch22/3
  Delay35/1 -> Switch11/3
  Delay13/1 -> Switch21/3
  Delay29/1 -> Switch10/3
  Delay27/1 -> Switch8/3
  Delay20/1 -> Switch3/3
  Delay22/1 -> Switch4/3

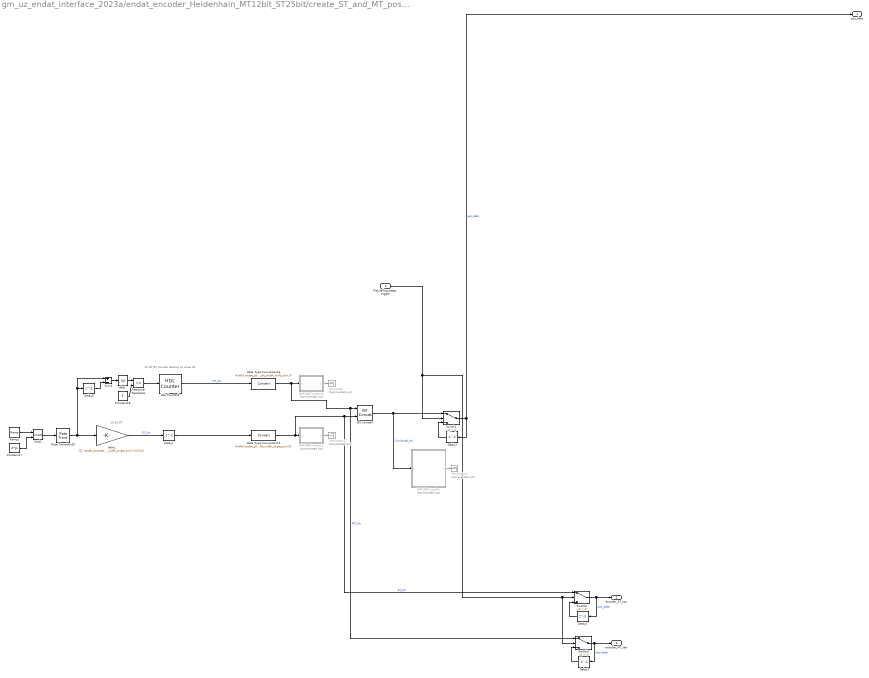
== system gm_uz_endat_interface_2023a/endat_encoder_Heidenhain_MT12bit_ST25bit/create_ST_and_MT_position_values ==
  note: 25 bit ST
  note: 12 bit MT counter starting at value 42
  first_falling_edge_trigger : Inport
  Abs1 : Abs  SaturateOnIntegerOverflow=off
  Bit Concat4 : hdlsllib/Logic and Bit Operations/Bit Concat  numInputs=2
  Constant17 : Constant  Value=2*pi  SampleTime=t_clock
  Constant18 : Constant  Value=5  SampleTime=t_clock
  Data Type Conversion12 : DataTypeConversion  OutDataTypeStr=fixdt(0,endat_encoder_bit_width_single_turn,0)  SaturateOnIntegerOverflow=off  RndMeth=Floor
  Data Type Conversion13 : DataTypeConversion  OutDataTypeStr=fixdt(0,endat_encoder_bit_width_multi_turn,0)  SaturateOnIntegerOverflow=off  RndMeth=Floor
  Delay{1..3,6..7} (5 alike) : Delay  DelayLength=1
  Gain1 : Gain  Gain=((2^endat_encoder_bit_width_single_turn)-1)/(2*pi)  OutDataTypeStr=uint32
  HDL Counter3 : hdlsllib/Sources/HDL Counter  CountType=Count limited  CountInit=42  CountStep=1  CountMax=4095  CountFromType=Initial value  CountFrom=42  CountResetPort=off  CountLoadPort=off  CountEnbPort=on  CountDirPort=off  CountHitOutputPort=off  CountDataType=Unsigned  CountWordLen=12  CountFracLen=0  CountSampTime=1
  MATLAB Function : MATLAB Function  Commented=on  TreatAsAtomicUnit=on
  MATLAB Function1 : MATLAB Function  Commented=on  TreatAsAtomicUnit=on
  MATLAB Function2 : MATLAB Function  Commented=on  TreatAsAtomicUnit=on
  Mod1 : Math  Operator=mod
  Ramp1 : simulink/Sources/Ramp  slope=2*pi*50  start=0  InitialOutput=0
  Rate Transition20 : RateTransition  OutPortSampleTime=t_clock
  Relational Operator6 : RelationalOperator  OutDataTypeStr=boolean  RndMeth=Simplest  InputSameDT=off
  Sum1 : Sum  Inputs=+-
  Switch1 : Switch  Criteria=u2 > Threshold  SaturateOnIntegerOverflow=off  InputSameDT=off
  Switch2 : Switch  Criteria=u2 > Threshold  SaturateOnIntegerOverflow=off  InputSameDT=off
  Switch3 : Switch  Criteria=u2 > Threshold  SaturateOnIntegerOverflow=off  InputSameDT=off
  Terminator : Terminator  Commented=on
  Terminator1 : Terminator  Commented=on
  Terminator2 : Terminator  Commented=on
  pos_data : Outport
  encoder_ST_raw : Outport  Port=2
  encoder_MT_raw : Outport  Port=3
  wires:
  Delay3/1 -> Switch3/3
  Switch3/1 -> Delay3/1, encoder_MT_raw/1  "pos_data"
  first_falling_edge_trigger/1 -> Switch1/2, Switch2/2, Switch3/2
  Delay1/1 -> Switch2/3
  Switch2/1 -> Delay1/1, encoder_ST_raw/1  "pos_data"
  MATLAB Function/1(y) -> Terminator2/1
  MATLAB Function1/1(y) -> Terminator1/1
  Mod1/1 -> Rate Transition20/1
  Gain1/1 -> Delay7/1  "ST_bin"
  Sum1/1 -> Abs1/1
  Abs1/1 -> Relational Operator6/1
  Delay6/1 -> Sum1/2
  Delay2/1 -> Switch1/3
  Relational Operator6/1 -> HDL Counter3/1
  Data Type Conversion13/1 -> MATLAB Function2/1(u), Bit Concat4/1, Switch3/1  "MT_bin"
  Ramp1/1 -> Mod1/1
  Bit Concat4/1 -> MATLAB Function/1(u), Switch1/1  "Combined_bin"
  HDL Counter3/1 -> Data Type Conversion13/1  "MT_bin"
  Switch1/1 -> Delay2/1, pos_data/1  "pos_data"
  Rate Transition20/1 -> Gain1/1, Delay6/1, Sum1/1
  Delay7/1 -> Data Type Conversion12/1
  Constant18/1 -> Relational Operator6/2
  Data Type Conversion12/1 -> MATLAB Function1/1(u), Bit Concat4/2, Switch2/1  "ST_bin"
  Constant17/1 -> Mod1/2
  MATLAB Function2/1(y) -> Terminator/1

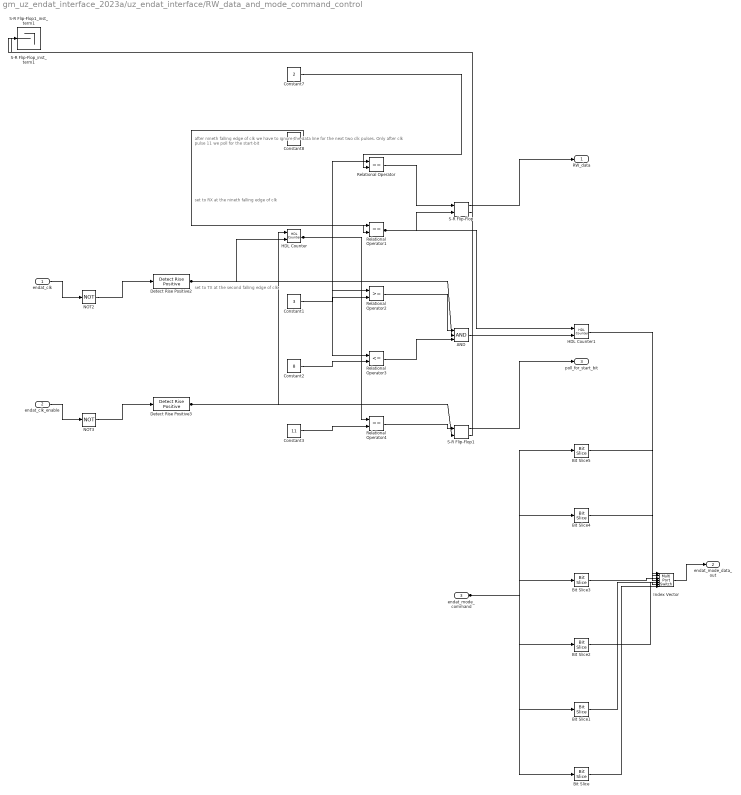
== system gm_uz_endat_interface_2023a/uz_endat_interface/RW_data_and_mode_command_control ==
  note: after nineth falling edge of clk we have to ignore the data line for the next two clk pulses. Only after clk pulse 11 we poll for the start-bit
  note: set to RX at the nineth falling edge of clk
  note: set to TX at the second falling edge of clk
  endat_clk : Inport  OutDataTypeStr=boolean  PortDimensions=1  SampleTime=1e-08
  endat_clk_enable : Inport  Port=2  OutDataTypeStr=boolean  PortDimensions=1  SampleTime=1e-08
  endat_mode_command : Inport  Port=3  OutDataTypeStr=uint32  PortDimensions=1  SampleTime=1e-08
  AND : Logic  Inputs=3  AllPortsSameDT=off  OutDataTypeStr=boolean  SampleTime=1e-08
  Bit Slice : hdlsllib/Logic and Bit Operations/Bit Slice  lidx=double(0)  ridx=double(0)
  Bit Slice1 : hdlsllib/Logic and Bit Operations/Bit Slice  lidx=double(1)  ridx=double(1)
  Bit Slice2 : hdlsllib/Logic and Bit Operations/Bit Slice  lidx=double(2)  ridx=double(2)
  Bit Slice3 : hdlsllib/Logic and Bit Operations/Bit Slice  lidx=double(3)  ridx=double(3)
  Bit Slice4 : hdlsllib/Logic and Bit Operations/Bit Slice  lidx=double(4)  ridx=double(4)
  Bit Slice5 : hdlsllib/Logic and Bit Operations/Bit Slice  lidx=double(5)  ridx=double(5)
  Constant1 : Constant  Value=3  OutDataTypeStr=uint8  SampleTime=1e-08
  Constant2 : Constant  Value=8  OutDataTypeStr=uint8  SampleTime=1e-08
  Constant3 : Constant  Value=11  OutDataTypeStr=uint8  SampleTime=1e-08
  Constant7 : Constant  Value=2  OutDataTypeStr=uint8  SampleTime=1e-08
  Constant8 : Constant  Value=9  OutDataTypeStr=uint8  SampleTime=1e-08
  Detect Rise Positive2 : simulink/Logic and Bit Operations/Detect Rise Positive  vinit=0  OutDataTypeStr=boolean
  Detect Rise Positive3 : simulink/Logic and Bit Operations/Detect Rise Positive  vinit=0  OutDataTypeStr=boolean
  HDL Counter : hdlsllib/Sources/HDL Counter  CountType=Free running  CountInit=0  CountStep=1  CountMax=25  CountFromType=Initial value  CountFrom=0  CountResetPort=on  CountLoadPort=off  CountEnbPort=on  CountDirPort=off  CountHitOutputPort=off  CountDataType=Unsigned  CountWordLen=8  CountFracLen=0  CountSampTime=1
  HDL Counter1 : hdlsllib/Sources/HDL Counter  CountType=Count limited  CountInit=0  CountStep=1  CountMax=5  CountFromType=Initial value  CountFrom=0  CountResetPort=on  CountLoadPort=off  CountEnbPort=on  CountDirPort=off  CountHitOutputPort=off  CountDataType=Unsigned  CountWordLen=8  CountFracLen=0  CountSampTime=1
  Index Vector : MultiPortSwitch  DataPortOrder=Zero-based contiguous  Inputs=6  DiagnosticForDefault=None  zeroidx=on  OutDataTypeStr=fixdt(0, 1, 0)  SampleTime=1e-08  SaturateOnIntegerOverflow=off  InputSameDT=off
  NOT2 : Logic  Operator=NOT  Inputs=1  AllPortsSameDT=off  OutDataTypeStr=boolean  SampleTime=1e-08
  NOT3 : Logic  Operator=NOT  Inputs=1  AllPortsSameDT=off  OutDataTypeStr=boolean  SampleTime=1e-08
  Relational Operator : RelationalOperator  Operator===  OutDataTypeStr=boolean  SampleTime=1e-08  InputSameDT=off
  Relational Operator1 : RelationalOperator  Operator===  OutDataTypeStr=boolean  SampleTime=1e-08  InputSameDT=off
  Relational Operator2 : RelationalOperator  OutDataTypeStr=boolean  SampleTime=1e-08  InputSameDT=off
  Relational Operator3 : RelationalOperator  Operator=<=  OutDataTypeStr=boolean  SampleTime=1e-08  InputSameDT=off
  Relational Operator4 : RelationalOperator  Operator===  OutDataTypeStr=boolean  SampleTime=1e-08  InputSameDT=off
  S-R Flip-Flop : simulink_extras/Flip Flops/S-R Flip-Flop  initial_condition=0
  S-R Flip-Flop1 : simulink_extras/Flip Flops/S-R Flip-Flop  initial_condition=0
  S-R Flip-Flop1_inst_term1 : Terminator
  S-R Flip-Flop_inst_term1 : Terminator
  RW_data : Outport  SampleTime=1e-08
  endat_mode_data_out : Outport  Port=2  SampleTime=1e-08
  poll_for_start_bit : Outport  Port=3  SampleTime=1e-08
  wires:
  AND/1 -> HDL Counter1/2
  Bit Slice/1 -> Index Vector/7
  Bit Slice1/1 -> Index Vector/6
  Bit Slice2/1 -> Index Vector/5
  Bit Slice3/1 -> Index Vector/4
  Bit Slice4/1 -> Index Vector/3
  Bit Slice5/1 -> Index Vector/2
  Constant1/1 -> Relational Operator2/2
  Constant2/1 -> Relational Operator3/2
  Constant3/1 -> Relational Operator4/2
  Constant7/1 -> Relational Operator/2
  Constant8/1 -> Relational Operator1/2
  Detect Rise Positive2/1 -> AND/2, HDL Counter/2
  Detect Rise Positive3/1 -> S-R Flip-Flop1/2, HDL Counter/1
  HDL Counter/1 -> Relational Operator4/1, Relational Operator3/1, Relational Operator2/1, Relational Operator1/1, Relational Operator/1
  HDL Counter1/1 -> Index Vector/1
  Index Vector/1 -> endat_mode_data_out/1
  NOT2/1 -> Detect Rise Positive2/1
  NOT3/1 -> Detect Rise Positive3/1
  Relational Operator/1 -> S-R Flip-Flop/1
  Relational Operator1/1 -> HDL Counter1/1, S-R Flip-Flop/2
  Relational Operator2/1 -> AND/1
  Relational Operator3/1 -> AND/3
  Relational Operator4/1 -> S-R Flip-Flop1/1
  S-R Flip-Flop/1 -> RW_data/1
  S-R Flip-Flop/2 -> S-R Flip-Flop_inst_term1/1
  S-R Flip-Flop1/1 -> poll_for_start_bit/1
  S-R Flip-Flop1/2 -> S-R Flip-Flop1_inst_term1/1
  endat_clk/1 -> NOT2/1
  endat_clk_enable/1 -> NOT3/1
  endat_mode_command/1 -> Bit Slice5/1, Bit Slice4/1, Bit Slice3/1, Bit Slice2/1, Bit Slice1/1, Bit Slice/1
